simulink model "FM_V6_Zikun"  (R2022b)
settings: Solver=VariableStepAuto  StartTime=0.0  StopTime=1240
values from neighbouring files (symbols this model uses):
  A_fc = 550    [CNV.m]
  A_st = 1.1*A_fc*1E-4*n_cell*0.0012    (= 0.047553)    [CNV.m]
  A_T_rm = 0.005    [CNV.m]
  b11 = 0.005139    [CNV.m]
  b12 = 0.00326    [CNV.m]
  b2 = 350    [CNV.m]
  c1 = 10    [CNV.m]
  c3 = 2    [CNV.m]
  cc = 30    [CNV.m]
  Cd_rm = 0.0124    [CNV.m]
  Cp_air = 1005    [CNV.m]
  Cp_cl = 4180    [CNV.m]
  Cp_st = Cp_Al*1.5    (= 1350)    [CNV.m]
  F = 96485    [CNV.m]
  gamma = 1.4    [CNV.m]
  H_conv_st = 3    [CNV.m]
  i_max = 2.2    [CNV.m]
  k_ca_out = 0.2177*10^(-5)    (= 2.177e-06)    [CNV.m]
  K_sm_out = 0.3629*10^-5    (= 3.629e-06)    [CNV.m]
  kd_cp = 0.01    [CNV.m]
  kd_rm = 0    [CNV.m]
  ki_cp = 0.1    [CNV.m]
  ki_fan = -1E-5    (= -1e-05)    [CNV.m]
  ki_rm = -5E-8    (= -5e-08)    [CNV.m]
  kp_cp = 7.5    [CNV.m]
  kp_fan = -0.5    [CNV.m]
  kp_rm = -8E-7    (= -8e-07)    [CNV.m]
  M_a = 29*10^-3    (= 0.029)    [CNV.m]
  M_H2 = 2*10^-3    (= 0.002)    [CNV.m]
  m_H2_initial = P_atm*V_an/(R_H2*T_atm)    (= 0.00044494386048)    [CNV.m]
  m_H2O_initial = 0.005    [CNV.m]
  M_m_dry = 1.1    [CNV.m]
  M_N2 = 28*10^-3    (= 0.028)    [CNV.m]
  m_N2_initial = P_atm*(1-y_O2)*V_ca/(R_N2*T_atm)    (= 0.00586138039643)    [CNV.m]
  M_O2 = 32*10^-3    (= 0.032)    [CNV.m]
  m_O2_initial = P_atm*y_O2*V_ca/(R_O2*T_atm)    (= 0.00177998712422)    [CNV.m]
  m_st = n_cell*A_fc*t_m*rho_m_dry+(V_ca+V_an)*rho_Al*2.5    (= 87.4506875)    [CNV.m]
  M_v = 18*10^-3    (= 0.018)    [CNV.m]
  n_cell = 655    [CNV.m]
  P_a = P_atm*(1-L*h/T_atm)^(g*M_a/(R*L))    [CNV.m]
  P_atm = 101.25*10^3    (= 101250)    [CNV.m]
  P_ca_ref = 2.5*P_a    [CNV.m]
  phi_a = 0.1    [CNV.m]
  phi_des = 1    [CNV.m]
  R = 8.315    [CNV.m]
  R_a = 286.9    [CNV.m]
  R_H2 = 4124.3    [CNV.m]
  R_N2 = 296.8    [CNV.m]
  R_O2 = 259.8    [CNV.m]
  R_v = 461.5    [CNV.m]
  rho_a = P_a/(R_a*T_a)    [CNV.m]
  rho_H2 = 0.0899    [CNV.m]
  rho_m_dry = 0.002    [CNV.m]
  rho_N2 = 1.165    [CNV.m]
  T_a = T_atm-h*L    [CNV.m]
  T_atm = 298.15    [CNV.m]
  T_cl = 353.15    [CNV.m]
  t_m = 0.01    [CNV.m]
  T_rm = 303.15    [CNV.m]
  T_st_ref = 353.15    [CNV.m]
  V_an = n_cell*A_fc*10^(-4)*0.0005*0.3    (= 0.00540375)    [CNV.m]
  V_ca = n_cell*A_fc*10^(-4)*0.0006*0.3    (= 0.0064845)    [CNV.m]
  V_rm = 0.005    [CNV.m]
  V_sm = 0.02    [CNV.m]
  y_O2_ca_in = 0.21    [CNV.m]
libraries: fl_lib x64, nesl_utility x40, ee_lib x18, fl_ps_legacy_lib x6, SimscapeFluids_lib x5, slpidlib x4, simulink x3, batteryecm_lib x1, autolibshared x1
(part 3 of 6)

== system FM_V6_Zikun/Subsystem/Air Cooler ==
  W_sm_out : Inport
  P_sm : Inport  Port=2
  Constant : Constant  Value=P_a
  Constant1 : Constant  Value=T_a
  Constant2 : Constant  Value=phi_a
  Constant3 : Constant  Value=T_cl
  MATLAB Function : MATLAB Function  TreatAsAtomicUnit=on
  W_cl : Outport
  phi_cl : Outport  Port=2
  psat_Tcl : Outport  Port=3
  P_cl : Outport  Port=4
  T_cl : Outport  Port=5
  wires:
  P_sm/1 -> P_cl/1, MATLAB Function/1(P_cl)
  MATLAB Function/1(phi_cl) -> phi_cl/1
  MATLAB Function/2(T_cl) -> T_cl/1
  W_sm_out/1 -> W_cl/1
  MATLAB Function/3(psat_Tcl) -> psat_Tcl/1
  Constant/1 -> MATLAB Function/2(P_a)
  Constant1/1 -> MATLAB Function/3(T_a)
  Constant2/1 -> MATLAB Function/4(phi_a)
  Constant3/1 -> MATLAB Function/5("T_cl ")

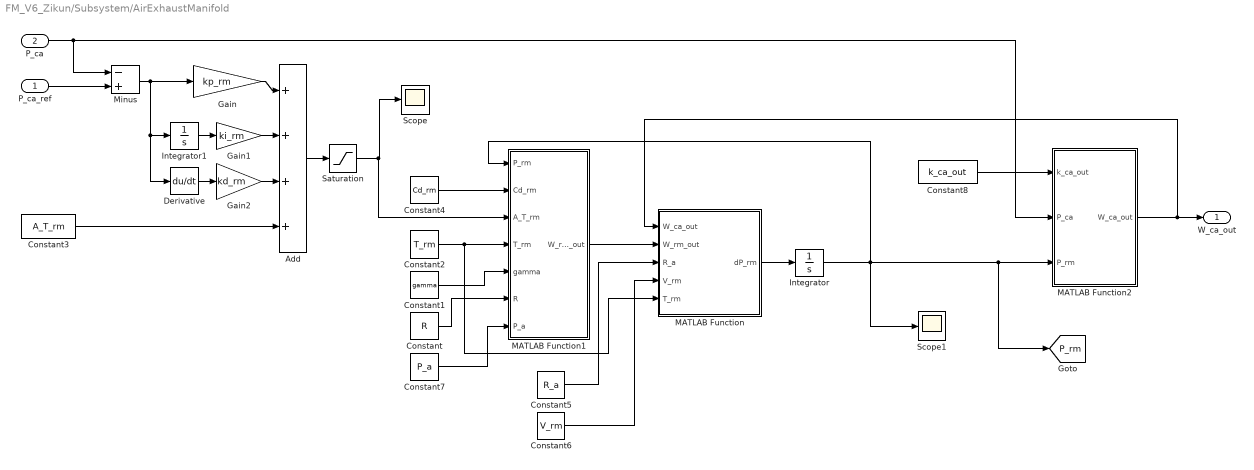
== system FM_V6_Zikun/Subsystem/AirExhaustManifold ==
  P_ca_ref : Inport
  P_ca : Inport  Port=2
  Add : Sum  Inputs=++++
  Constant : Constant  Value=R
  Constant1 : Constant  Value=gamma
  Constant2 : Constant  Value=T_rm
  Constant3 : Constant  Value=A_T_rm
  Constant4 : Constant  Value=Cd_rm
  Constant5 : Constant  Value=R_a
  Constant6 : Constant  Value=V_rm
  Constant7 : Constant  Value=P_a
  Constant8 : Constant  Value=k_ca_out
  Derivative : Derivative
  Gain : Gain  Gain=kp_rm
  Gain1 : Gain  Gain=ki_rm
  Gain2 : Gain  Gain=kd_rm
  Integrator : Integrator  InitialCondition=P_atm
  Integrator1 : Integrator
  MATLAB Function : MATLAB Function  TreatAsAtomicUnit=on
  MATLAB Function1 : MATLAB Function  TreatAsAtomicUnit=on
  MATLAB Function2 : MATLAB Function  TreatAsAtomicUnit=on
  Minus : Sum  Inputs=-+
  Saturation : Saturate  UpperLimit=0.04  LowerLimit=0
  Scope : Scope
  Scope1 : Scope
  W_ca_out : Outport
  tag scope: P_rm=global
  wires:
  MATLAB Function1/1(W_rm_out) -> MATLAB Function/2(W_rm_out)
  MATLAB Function/1(dP_rm) -> Integrator/1
  Integrator/1 -> Scope1/1, [P_rm], MATLAB Function2/3(P_rm), MATLAB Function1/1(P_rm)
  Constant/1 -> MATLAB Function1/6(R)
  Constant1/1 -> MATLAB Function1/5(gamma)
  Constant2/1 -> MATLAB Function/5(T_rm), MATLAB Function1/4(T_rm)
  Constant4/1 -> MATLAB Function1/2(Cd_rm)
  Constant5/1 -> MATLAB Function/3(R_a)
  Constant6/1 -> MATLAB Function/4(V_rm)
  Constant7/1 -> MATLAB Function1/7(P_a)
  MATLAB Function2/1(W_ca_out) -> MATLAB Function/1(W_ca_out), W_ca_out/1
  P_ca/1 -> Minus/1, MATLAB Function2/2(P_ca)
  Constant8/1 -> MATLAB Function2/1(k_ca_out)
  P_ca_ref/1 -> Minus/2
  Minus/1 -> Derivative/1, Integrator1/1, Gain/1
  Integrator1/1 -> Gain1/1
  Gain/1 -> Add/1
  Gain1/1 -> Add/2
  Constant3/1 -> Add/4
  Derivative/1 -> Gain2/1
  Gain2/1 -> Add/3
  Add/1 -> Saturation/1
  Saturation/1 -> MATLAB Function1/3(A_T_rm), Scope/1

== system FM_V6_Zikun/Subsystem/Blower ==
  P_an_in : Inport
  lambda_H2 : Inport  Port=2
  ny_blower : Inport  Port=3
  W_H2_tank : Inport  Port=4
  P_an : Inport  Port=5
  H2_ratio : Inport  Port=6
  Constant : Constant  Value=rho_H2
  Constant1 : Constant  Value=rho_N2
  MATLAB Function : MATLAB Function  TreatAsAtomicUnit=on
  W_an_in : Outport
  W_an_out : Outport  Port=2
  P_blower : Outport  Port=3
  wires:
  lambda_H2/1 -> MATLAB Function/4(lambda_H2)
  H2_ratio/1 -> MATLAB Function/6(H2_ratio)
  ny_blower/1 -> MATLAB Function/5(ny_blower)
  W_H2_tank/1 -> MATLAB Function/3(W_H2_tank)
  Constant/1 -> MATLAB Function/2(rho_N2)
  Constant1/1 -> MATLAB Function/1(rho_H2)
  MATLAB Function/1(W_an_in) -> W_an_in/1
  MATLAB Function/2(W_an_out) -> W_an_out/1
  MATLAB Function/3(P_blower) -> P_blower/1
  P_an/1 -> MATLAB Function/8(P_an)
  P_an_in/1 -> MATLAB Function/7(P_an_in)

== system FM_V6_Zikun/Subsystem/Compressor ==
  I_st : Inport
  P_ca : Inport  Port=2
  P_sm : Inport  Port=3
  Abs : Abs  ZeroCross=off  SaturateOnIntegerOverflow=off
  Add : Sum  Inputs=+-
  Constant2 : Constant
  Constant6 : Constant  Value=T_a
  Constant7 : Constant  Value=P_a
  Display : Display
  Divide : Product  Inputs=*/
  Divide1 : Product  Inputs=**
  Power calc 2 : Subsystem
      settings: PortSchema="{\"entries\":[{\"content\":{\"sides\":[{\"content\":{\"connectorIds\":[\"In1\",\"In2\",\"In3\"]},\"type\":\"ConnectorPlacement.EquallySpacedRectSide\",\"uuid\":\"8b079436-ea2a-4c47-8bc6-4d08a6a8278c\"},{\"content\":{\"connectorIds\":[\"In4\",\"Out1\"],\"side\":\"RIGHT\"},\"type\":\"ConnectorPlacement.EquallySpacedRectSide\",\"uuid\":\"2ad3baf7-33f6-4d58-a512-a1947502cd3d\"},{\"content\":{\"connectorIds\":[],\"side\":\"TOP\"},\"type\":\"ConnectorPlacement.EquallySpacedRectSide\",\"uuid\":\"d6297fa1-7292-4bed-8060-dba2913c02c2\"}]},\"type\":\"ConnectorPlacement.EquallySpacedConnector\",\"uuid\":\"103abd89-9500-4b01-83b0-a840418a3fc8\"}],\"packageUris\":[\"http://schema.mathworks.com/mf0/Connector/R2020b\"],\"version\":\"1.0\"}"
  Saturation : Saturate  UpperLimit=0.2  LowerLimit=4e-3  ZeroCross=off
  Scope : Scope
  Scope1 : Scope
  Subsystem : Subsystem
  Temperature of the air leaving the compressor (2.8) : Subsystem
  maximum efficiency of compressor : Constant  Value=0.9
  "rate of specific heats of air " : Constant  Value=gamma
  W_cp : Outport
  T_cp_out : Outport  Port=2
  Power_cp_them : Outport  Port=3
  Power_cp_tot : Outport  Port=4
  wires:
  "rate of specific heats of air "/1 -> Power calc 2/3(gamma), Temperature of the air leaving the compressor (2.8)/5(gamma)
  Constant6/1 -> Temperature of the air leaving the compressor (2.8)/1(T_atm)
  maximum efficiency of compressor/1 -> Add/2, Divide/2, Temperature of the air leaving the compressor (2.8)/2(eta_cp)
  Temperature of the air leaving the compressor (2.8)/1(T_cp_out) -> T_cp_out/1
  Constant7/1 -> Power calc 2/2(P_cp_in), Temperature of the air leaving the compressor (2.8)/4(P_atm)
  I_st/1 -> Subsystem/2(I_st)
  Power calc 2/1(Power_cp) -> Divide/1
  Divide/1 -> Abs/1
  Constant2/1 -> Add/1
  Add/1 -> Divide1/2
  Divide1/1 -> Power_cp_them/1
  Abs/1 -> Divide1/1, Display/1, Power_cp_tot/1
  [W_O2_ca_in] -> Subsystem/1(W_O2_ca_in)
  P_ca/1 -> Subsystem/3(P_ca)
  P_sm/1 -> Power calc 2/1(P_cp_out), Temperature of the air leaving the compressor (2.8)/3(P_sm)
  Subsystem/1(W_cp) -> Saturation/1
  Saturation/1 -> Scope/1, W_cp/1, Scope1/1, Power calc 2/4(W_cp_in)

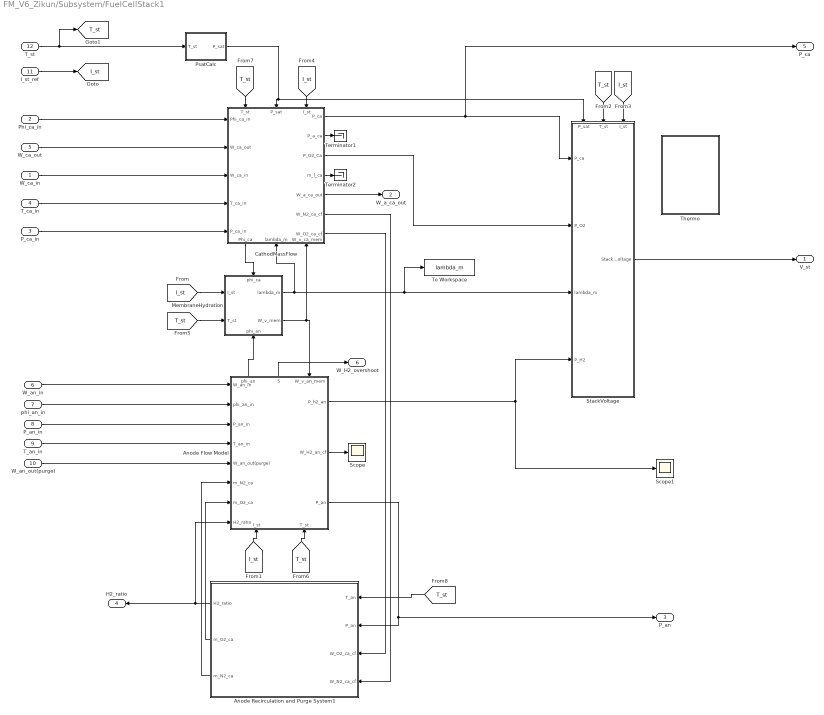
== system FM_V6_Zikun/Subsystem/FuelCellStack1 ==
  W_ca_in : Inport
  Phi_ca_in : Inport  Port=2
  P_ca_in : Inport  Port=3
  T_ca_in : Inport  Port=4
  W_ca_out : Inport  Port=5
  W_an_in : Inport  Port=6
  phi_an_in : Inport  Port=7
  P_an_in : Inport  Port=8
  T_an_in : Inport  Port=9
  W_an_out(purge) : Inport  Port=10
  I_st_ref : Inport  Port=11
  T_st : Inport  Port=12
  Anode Flow Model : Subsystem
      settings: PortSchema="{\"entries\":[{\"content\":{\"sides\":[{\"content\":{\"connectorIds\":[\"In1\",\"In2\",\"In3\",\"In4\",\"In5\",\"In6\",\"In7\",\"In8\"]},\"type\":\"ConnectorPlacement.EquallySpacedRectSide\",\"uuid\":\"477fe13c-ae2c-434a-aa62-6a7137066034\"},{\"content\":{\"connectorIds\":[\"Out1\",\"Out2\",\"Out3\"],\"side\":\"RIGHT\"},\"type\":\"ConnectorPlacement.EquallySpacedRectSide\",\"uuid\":\"66550877-05b9-4d53-a95b-0d13dddd1ae9\"},{\"content\":{\"connectorIds\":[\"Out4\",\"Out5\",\"In9\"],\"side\":\"TOP\"},\"type\":\"ConnectorPlacement.EquallySpacedRectSide\",\"uuid\":\"dee2e959-3be9-4270-9608-f17df99829af\"},{\"content\":{\"connectorIds\":[\"In10\",\"In11\"],\"side\":\"BOTTOM\"},\"type\":\"ConnectorPlacement.EquallySpacedRectSide\",\"uuid\":\"e68932cb-a3ca-49aa-99ac-394e109cb21d\"}]},\"type\":\"ConnectorPlacement.EquallySpacedConnector\",\"uuid\":\"e53fddc6-f473-4a61-b934-687e83f91b65\"}],\"packageUris\":[\"http://schema.mathworks.com/mf0/Connector/R2020b\"],\"version\":\"1.0\"}"
  Anode Recirculation and Purge System1 : Subsystem
      settings: PortSchema="{\"entries\":[{\"content\":{\"sides\":[{\"content\":{\"connectorIds\":[\"Out1\",\"Out2\",\"Out3\"]},\"type\":\"ConnectorPlacement.EquallySpacedRectSide\",\"uuid\":\"a717ff69-9a06-432a-8ec9-0b41de582fa8\"},{\"content\":{\"connectorIds\":[\"In1\",\"In2\",\"In3\",\"In4\"],\"side\":\"RIGHT\"},\"type\":\"ConnectorPlacement.EquallySpacedRectSide\",\"uuid\":\"e2c7096e-75de-462f-89fb-70e142ee793c\"},{\"content\":{\"connectorIds\":[],\"side\":\"TOP\"},\"type\":\"ConnectorPlacement.EquallySpacedRectSide\",\"uuid\":\"2426b314-6327-4045-9254-2b33a242dd4e\"},{\"content\":{\"connectorIds\":[],\"side\":\"BOTTOM\"},\"type\":\"ConnectorPlacement.EquallySpacedRectSide\",\"uuid\":\"28581630-fccf-4c59-a85b-fca9f25db1df\"}]},\"type\":\"ConnectorPlacement.EquallySpacedConnector\",\"uuid\":\"c799c0e9-037d-437b-b392-b2fa1dfcad00\"}],\"packageUris\":[\"http://schema.mathworks.com/mf0/Connector/R2020b\"],\"version\":\"1.0\"}"
  CathodMassFlow : Subsystem
      settings: PortSchema="{\"entries\":[{\"content\":{\"sides\":[{\"content\":{\"connectorIds\":[\"In1\",\"In2\",\"In3\",\"In4\",\"In5\"]},\"type\":\"ConnectorPlacement.EquallySpacedRectSide\",\"uuid\":\"a5816526-b2df-4ff7-b309-d39278f05798\"},{\"content\":{\"connectorIds\":[\"Out1\",\"Out2\",\"Out3\",\"Out4\",\"Out5\",\"Out6\",\"Out7\"],\"side\":\"RIGHT\"},\"type\":\"ConnectorPlacement.EquallySpacedRectSide\",\"uuid\":\"a3a8a0b8-4f26-4d97-8833-d547d26a82ce\"},{\"content\":{\"connectorIds\":[\"In6\",\"In7\",\"In8\"],\"side\":\"TOP\"},\"type\":\"ConnectorPlacement.EquallySpacedRectSide\",\"uuid\":\"a0145b7a-873e-4436-80c5-f848de3e3117\"},{\"content\":{\"connectorIds\":[\"Out8\",\"In9\",\"In10\"],\"side\":\"BOTTOM\"},\"type\":\"ConnectorPlacement.EquallySpacedRectSide\",\"uuid\":\"3c36750c-8b40-4a1a-a95d-a988a8ace63a\"}]},\"type\":\"ConnectorPlacement.EquallySpacedConnector\",\"uuid\":\"934b3933-c5aa-40b8-8fa9-71f43b151d81\"}],\"packageUris\":[\"http://schema.mathworks.com/mf0/Connector/R2020b\"],\"version\":\"1.0\"}"
  MembraneHydration : Subsystem
      settings: PortSchema="{\"entries\":[{\"content\":{\"sides\":[{\"content\":{\"connectorIds\":[\"In1\",\"In2\"]},\"type\":\"ConnectorPlacement.EquallySpacedRectSide\",\"uuid\":\"3fc204c3-9c69-492e-9375-472aea363e1b\"},{\"content\":{\"connectorIds\":[\"Out1\",\"Out2\"],\"side\":\"RIGHT\"},\"type\":\"ConnectorPlacement.EquallySpacedRectSide\",\"uuid\":\"92fcb20f-c63d-4632-a8b2-72361d3984f2\"},{\"content\":{\"connectorIds\":[\"In3\"],\"side\":\"TOP\"},\"type\":\"ConnectorPlacement.EquallySpacedRectSide\",\"uuid\":\"2bf67bc3-afc1-4ec2-8a6f-f1995431a2a1\"},{\"content\":{\"connectorIds\":[\"In4\"],\"side\":\"BOTTOM\"},\"type\":\"ConnectorPlacement.EquallySpacedRectSide\",\"uuid\":\"b4bf2ddb-e361-4582-99a1-8ca6e4cff378\"}]},\"type\":\"ConnectorPlacement.EquallySpacedConnector\",\"uuid\":\"9ca90662-d7f0-47d0-8eb8-23aab38cb896\"}],\"packageUris\":[\"http://schema.mathworks.com/mf0/Connector/R2020b\"],\"version\":\"1.0\"}"
  PsatCalc : MATLAB Function  TreatAsAtomicUnit=on
  Scope : Scope
  Scope1 : Scope
  StackVoltage : Subsystem
      settings: PortSchema="{\"entries\":[{\"content\":{\"sides\":[{\"content\":{\"connectorIds\":[\"In1\",\"In2\",\"In3\",\"In4\"]},\"type\":\"ConnectorPlacement.EquallySpacedRectSide\",\"uuid\":\"31c21434-8ccd-4c9e-84e7-d59d7b2b32c9\"},{\"content\":{\"connectorIds\":[\"Out1\"],\"side\":\"RIGHT\"},\"type\":\"ConnectorPlacement.EquallySpacedRectSide\",\"uuid\":\"a03264e4-aeb3-4f9b-a3b2-cfddd05e7880\"},{\"content\":{\"connectorIds\":[\"In5\",\"In6\",\"In7\"],\"side\":\"TOP\"},\"type\":\"ConnectorPlacement.EquallySpacedRectSide\",\"uuid\":\"8542eea2-4f96-46a3-8a8b-d86d68868d64\"}]},\"type\":\"ConnectorPlacement.EquallySpacedConnector\",\"uuid\":\"2ea05213-dddc-4bd5-a30f-0985ad8bd6f4\"}],\"packageUris\":[\"http://schema.mathworks.com/mf0/Connector/R2020b\"],\"version\":\"1.0\"}"
  Terminator1 : Terminator
  Terminator2 : Terminator
  Thermo : Subsystem
  To Workspace : ToWorkspace  VariableName=lambda_m  SaveFormat=Timeseries  SampleTime=-1
  V_st : Outport
  W_a_ca_out : Outport  Port=2
  P_an : Outport  Port=3
  H2_ratio : Outport  Port=4
  P_ca : Outport  Port=5
  W_H2_overshoot : Outport  Port=6
  tag scope: I_st=global, T_st=global
  wires:
  CathodMassFlow/1(P_ca) -> P_ca/1, StackVoltage/1(P_ca)
  CathodMassFlow/3(P_O2_Ca) -> StackVoltage/2(P_O2)
  CathodMassFlow/8(Phi_ca) -> MembraneHydration/3(phi_ca)
  Anode Flow Model/4(phi_an) -> MembraneHydration/4(phi_an)
  MembraneHydration/2(W_v_mem) -> CathodMassFlow/10(W_v_ca_mem), Anode Flow Model/9(W_v_an_mem)
  MembraneHydration/1(lambda_m) -> CathodMassFlow/9(lambda_m), To Workspace/1, StackVoltage/3(lambda_m)
  Anode Flow Model/1(P_h2_an) -> StackVoltage/4(P_H2), Scope1/1
  CathodMassFlow/5(W_a_ca_out) -> W_a_ca_out/1
  W_ca_in/1 -> CathodMassFlow/3(W_ca_in)
  W_ca_out/1 -> CathodMassFlow/2(W_ca_out)
  Phi_ca_in/1 -> CathodMassFlow/1(Phi_ca_in)
  W_an_in/1 -> Anode Flow Model/1(W_an_in)
  phi_an_in/1 -> Anode Flow Model/2(phi_an_in)
  P_an_in/1 -> Anode Flow Model/3(P_an_in)
  T_an_in/1 -> Anode Flow Model/4(T_an_in)
  CathodMassFlow/2(P_a_ca) -> Terminator1/1
  CathodMassFlow/4(m_l_ca) -> Terminator2/1
  T_ca_in/1 -> CathodMassFlow/4(T_ca_in)
  P_ca_in/1 -> CathodMassFlow/5(P_ca_in)
  T_st/1 -> [T_st], PsatCalc/1(T_st)
  I_st_ref/1 -> [I_st]
  [I_st] -> MembraneHydration/1(I_st)
  [I_st] -> Anode Flow Model/10(I_st)
  [I_st] -> StackVoltage/7(I_st)
  [I_st] -> CathodMassFlow/8(I_st)
  [T_st] -> CathodMassFlow/6(T_st)
  [T_st] -> StackVoltage/6(T_st)
  [T_st] -> Anode Flow Model/11(T_st)
  [T_st] -> MembraneHydration/2(T_st)
  CathodMassFlow/6(W_N2_ca_cf) -> Anode Recirculation and Purge System1/4(W_N2_ca_cf)
  CathodMassFlow/7(W_O2_ca_cf) -> Anode Recirculation and Purge System1/3(W_O2_ca_cf)
  W_an_out(purge)/1 -> Anode Flow Model/5(W_an_out(purge))
  Anode Recirculation and Purge System1/1(H2_ratio) -> Anode Flow Model/8(H2_ratio), H2_ratio/1
  Anode Recirculation and Purge System1/3(m_N2_ca) -> Anode Flow Model/6(m_N2_ca)
  Anode Recirculation and Purge System1/2(m_O2_ca) -> Anode Flow Model/7(m_O2_ca)
  Anode Flow Model/2(W_H2_an_cf) -> Scope/1
  [T_st] -> Anode Recirculation and Purge System1/1(T_an)
  PsatCalc/1(P_sat) -> CathodMassFlow/7(P_sat), StackVoltage/5(P_sat)
  StackVoltage/1(StackVoltage) -> V_st/1
  Anode Flow Model/5(W_H2_overshoot) -> W_H2_overshoot/1
  Anode Flow Model/3(P_an) -> P_an/1, Anode Recirculation and Purge System1/2(P_an)

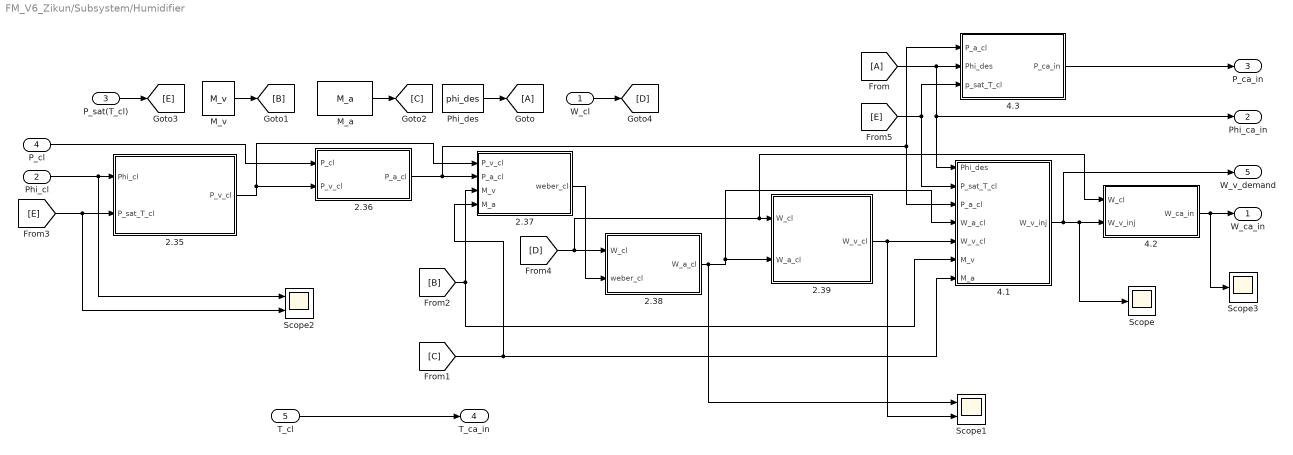
== system FM_V6_Zikun/Subsystem/Humidifier ==
  W_cl : Inport
  Phi_cl : Inport  Port=2
  P_sat(T_cl) : Inport  Port=3
  P_cl : Inport  Port=4
  T_cl : Inport  Port=5
  2.35 : MATLAB Function  TreatAsAtomicUnit=on
  2.36 : MATLAB Function  TreatAsAtomicUnit=on
  2.37 : MATLAB Function  TreatAsAtomicUnit=on
  2.38 : MATLAB Function  TreatAsAtomicUnit=on
  2.39 : MATLAB Function  TreatAsAtomicUnit=on
  4.1 : MATLAB Function  TreatAsAtomicUnit=on
  4.2 : MATLAB Function  TreatAsAtomicUnit=on
  4.3 : MATLAB Function  TreatAsAtomicUnit=on
  From : From
  Goto : Goto
  M_a : Constant  Value=M_a
  M_v : Constant  Value=M_v
  Phi_des : Constant  Value=phi_des
  Scope : Scope
  Scope1 : Scope  NumInputPorts=2
  Scope2 : Scope  NumInputPorts=2
  Scope3 : Scope
  W_ca_in : Outport
  Phi_ca_in : Outport  Port=2
  P_ca_in : Outport  Port=3
  T_ca_in : Outport  Port=4
  W_v_demand : Outport  Port=5
  wires:
  4.3/1(P_ca_in) -> P_ca_in/1
  4.1/1(W_v_inj) -> Scope/1, 4.2/2(W_v_inj), W_v_demand/1
  2.36/1(P_a_cl) -> 4.1/3(P_a_cl), 4.3/1(P_a_cl), 2.37/2(P_a_cl)
  2.39/1(W_v_cl) -> Scope1/2, 4.1/5(W_v_cl)
  2.38/1(W_a_cl) -> Scope1/1, 2.39/2(W_a_cl), 4.1/4(W_a_cl)
  2.35/1(P_v_cl) -> 2.37/1(P_v_cl), 2.36/2(P_v_cl)
  Phi_cl/1 -> Scope2/1, 2.35/1(Phi_cl)
  P_cl/1 -> 2.36/1(P_cl)
  Phi_des/1 -> Goto/1
  M_v/1 -> [B]
  M_a/1 -> [C]
  2.37/1(weber_cl) -> 2.38/2(weber_cl)
  P_sat(T_cl)/1 -> [E]
  [E] -> Scope2/2, 2.35/2(P_sat_T_cl)
  W_cl/1 -> [D]
  From/1 -> Phi_ca_in/1, 4.1/1(Phi_des), 4.3/2(Phi_des)
  [B] -> 4.1/6(M_v), 2.37/3(M_v)
  [C] -> 4.1/7(M_a), 2.37/4(M_a)
  [D] -> 4.2/1(W_cl), 2.39/1(W_cl), 2.38/1(W_cl)
  [E] -> 4.3/3(p_sat_T_cl), 4.1/2(P_sat_T_cl)
  T_cl/1 -> T_ca_in/1
  4.2/1(W_ca_in) -> Scope3/1, W_ca_in/1

== system FM_V6_Zikun/Subsystem/Hydrogen Tank // Hydrogen Valve // Regulator1 ==
  Tank Volume : Inport
  Initial Tank Pressure : Inport  Port=2
  Tank Temperature : Inport  Port=3
  Regulator Anode Pressure : Inport  Port=4
  P_an : Inport  Port=5
  Constant : Constant  Value=R_H2
  Gain : Gain  Gain=1/M_N2
  Integrator : Integrator
  MATLAB Function1 : MATLAB Function  TreatAsAtomicUnit=on
  PID Controller : slpidlib/PID Controller  Controller=PI  Form=Parallel  TimeDomain=Continuous-time  UseExternalTs=off  SampleTime=-1  IntegratorMethod=Forward Euler  FilterMethod=Forward Euler  ControllerParametersSource=internal  P=6e-7  I=0  UseKiTs=off  D=0  N=100  UseFilter=on  TunerSelectOption=Transfer Function Based (PID Tuner App)  InitialConditionSource=internal  InitialConditionForIntegrator=0  InitialConditionForFilter=0  DifferentiatorICPrevScaledInput=0  ExternalReset=none  TrackingMode=off  Kt=1  LimitOutput=on  SatLimitsSource=internal  UpperSaturationLimit=0.005  LowerSaturationLimit=-0.04  LinearizeAsGain=on  AntiWindupMode=none  Kb=1  LimitIntegrator=off  UpperIntegratorSaturationLimit=inf  LowerIntegratorSaturationLimit=-inf  POutMin=[]  POutMax=[]  IOutMin=[]  IOutMax=[]  DOutMin=[]  DOutMax=[]  NOutMin=[]  NOutMax=[]  SumOutMin=[]  SumOutMax=[]  SaturationOutMin=[]  SaturationOutMax=[]  PParamMin=[]  PParamMax=[]  IParamMin=[]  IParamMax=[]  DParamMin=[]  DParamMax=[]  NParamMin=[]  NParamMax=[]  KbParamMin=[]  KbParamMax=[]  KtParamMin=[]  KtParamMax=[]  KbOutMin=[]  KbOutMax=[]  KtOutMin=[]  KtOutMax=[]  IntegratorOutMin=[]  IntegratorOutMax=[]  FilterOutMin=[]  FilterOutMax=[]  SumI1OutMin=[]  SumI1OutMax=[]  SumI2OutMin=[]  SumI2OutMax=[]  SumI3OutMin=[]  SumI3OutMax=[]  SumI4OutMin=[]  SumI4OutMax=[]  SumDOutMin=[]  SumDOutMax=[]  DifferentiatorOutMin=[]  DifferentiatorOutMax=[]  FilterDiffOutCoefMin=[]  FilterDiffOutCoefMax=[]  ReciprocalOutMin=[]  ReciprocalOutMax=[]  SumDenOutMin=[]  SumDenOutMax=[]  SumNumOutMin=[]  SumNumOutMax=[]  DivideOutMin=[]  DivideOutMax=[]  UdiffTsProdOutMin=[]  UdiffTsProdOutMax=[]  NTsProdOutMin=[]  NTsProdOutMax=[]  UintegralTsProdOutMin=[]  UintegralTsProdOutMax=[]  UngainTsProdOutMin=[]  UngainTsProdOutMax=[]  ClampingZeroOutDataTypeStr=Inherit: Inherit via back propagation  ClampingZeroOutMin=[]  ClampingZeroOutMax=[]  FilterDenConstantOutDataTypeStr=Inherit: Inherit via back propagation  FilterDenConstantOutMin=[]  FilterDenConstantOutMax=[]  PCopyOutDataTypeStr=Inherit: Inherit via back propagation  PCopyOutMin=[]  PCopyOutMax=[]  NCopyOutDataTypeStr=Inherit: Inherit via back propagation  NCopyOutMin=[]  NCopyOutMax=[]  IntegratorContinuousStateAttributes=''  IntegratorStateMustResolveToSignalObject=off  IntegratorRTWStateStorageClass=Auto  FilterContinuousStateAttributes=''  FilterStateMustResolveToSignalObject=off  FilterRTWStateStorageClass=Auto  ParallelPVariant=InternalParameters  IdealPVariant=Disabled  IVariant=InternalParameters  DVariant=Disabled  IntegratorVariant=Continuous  SatVariant=Enabled  AWVariant=Passthrough  PCopyVariant=Disabled  TRVariant=Disabled  FdbkBlocksVariant=Forward  IdealPFdbkVariant=Disabled  SatFdbkVariant=Disabled  DerivativeFilterVariant=Disabled  NVariant=Disabled  NCopyVariant=Disabled_SignalSpec  FilterICVariant=Disabled  IntegratorICVariant=InternalICs  ExternalResetVariant=Disabled  TRSumVariant=Passthrough  SumFdbkVariant=Disabled  SumVariant=Sum_PI  TsampFilterVariant=InternalTs  TsampNgainVariant=Passthrough  TsampIntegralVariant=Passthrough  ExternalSaturationOutDataTypeStr=Inherit: Same as second input
  Scope : Scope
  Subtract : Sum  Inputs=+-
  P_tank : Outport
  W_H2_tank : Outport  Port=2
  wires:
  P_an/1 -> Subtract/2
  Regulator Anode Pressure/1 -> Subtract/1
  Integrator/1 -> Gain/1
  Gain/1 -> MATLAB Function1/5(n_consumed)
  Tank Volume/1 -> MATLAB Function1/2(V_tank)
  Tank Temperature/1 -> MATLAB Function1/3(T_tank)
  Initial Tank Pressure/1 -> MATLAB Function1/4(P_tank_nom)
  Constant/1 -> MATLAB Function1/1(R_H2)
  MATLAB Function1/1(P_tank) -> P_tank/1
  Subtract/1 -> PID Controller/1
  PID Controller/1 -> Scope/1, Integrator/1, W_H2_tank/1

== system FM_V6_Zikun/Subsystem/Subsystem ==
  W_H2_Tank : Inport
  P_an : Inport  Port=2
  Add : Sum  Inputs=+-
  Add1 : Sum  Inputs=+-
  Constant : Constant  Value=R_H2
  Constant1 : Constant  Value=T_a
  Constant2 : Constant  Value=1*10^-3
  Gain : Gain  Gain=1e-8
  Integrator : Integrator  InitialCondition=1e-4
  MATLAB Function : MATLAB Function  TreatAsAtomicUnit=on
  Scope : Scope
  Scope1 : Scope
  W_H2_manifold : Outport
  wires:
  Constant/1 -> MATLAB Function/2(R_H2)
  Constant1/1 -> MATLAB Function/3(T_rm)
  Constant2/1 -> MATLAB Function/4(V_H2_manifold)
  MATLAB Function/1(P_H2_manifold) -> Add/1
  P_an/1 -> Add/2
  Add/1 -> Gain/1
  Gain/1 -> Add1/2, Scope/1, W_H2_manifold/1
  Integrator/1 -> MATLAB Function/1(m_H2), Scope1/1
  W_H2_Tank/1 -> Add1/1
  Add1/1 -> Integrator/1

== system FM_V6_Zikun/Subsystem/Subsystem2 ==
  I_st : Inport
  P_st : Inport  Port=2
  Subsystem : Subsystem
  ThermoCalc : Subsystem
  T_st : Outport
  P_tot : Outport  Port=2
  P_fan_loss : Outport  Port=3
  P_pump_loss : Outport  Port=4
  wires:
  ThermoCalc/1(T_st) -> Subsystem/1(T_cl_in), T_st/1
  P_st/1 -> ThermoCalc/2(P_st)
  I_st/1 -> Subsystem/2(I_st), ThermoCalc/1(I_st)
  Subsystem/3(P_cl) -> ThermoCalc/3(P_cl)
  Subsystem/1(P_pump_loss) -> P_pump_loss/1
  Subsystem/2(P_fan_loss) -> P_fan_loss/1
  ThermoCalc/2(P_tot_st) -> P_tot/1

== system FM_V6_Zikun/Subsystem/Supply Manifold ==
  W_cp : Inport
  T_cp_out : Inport  Port=2
  P_ca : Inport  Port=3
  Manifold Filling : Subsystem
      settings: PortSchema="{\"entries\":[{\"content\":{\"sides\":[{\"content\":{\"connectorIds\":[\"In1\",\"In2\"]},\"type\":\"ConnectorPlacement.EquallySpacedRectSide\",\"uuid\":\"5b708061-f651-4e95-ab82-a4e5a10c41aa\"},{\"content\":{\"connectorIds\":[],\"side\":\"RIGHT\"},\"type\":\"ConnectorPlacement.EquallySpacedRectSide\",\"uuid\":\"45f2c177-5321-40a9-9b70-6a6ced21c730\"},{\"content\":{\"connectorIds\":[],\"side\":\"TOP\"},\"type\":\"ConnectorPlacement.EquallySpacedRectSide\",\"uuid\":\"ee9f469e-0be0-432d-ad01-7aba5a85248f\"},{\"content\":{\"connectorIds\":[\"Out1\",\"Out2\",\"In3\"],\"side\":\"BOTTOM\"},\"type\":\"ConnectorPlacement.EquallySpacedRectSide\",\"uuid\":\"36fd777e-57dd-45d2-bfa2-d5269b7bf5c5\"}]},\"type\":\"ConnectorPlacement.EquallySpacedConnector\",\"uuid\":\"e32288af-c3d9-443b-a6e9-38324f9252c2\"}],\"packageUris\":[\"http://schema.mathworks.com/mf0/Connector/R2020b\"],\"version\":\"1.0\"}"
  Nozzle : Subsystem
      settings: PortSchema="{\"entries\":[{\"content\":{\"sides\":[{\"content\":{\"connectorIds\":[\"In1\"]},\"type\":\"ConnectorPlacement.EquallySpacedRectSide\",\"uuid\":\"5777e37f-23fb-4f15-af78-9892d3d66602\"},{\"content\":{\"connectorIds\":[],\"side\":\"RIGHT\"},\"type\":\"ConnectorPlacement.EquallySpacedRectSide\",\"uuid\":\"6b20c729-b7c3-4bc6-b5e0-0939bc80540e\"},{\"content\":{\"connectorIds\":[\"In2\",\"Out1\"],\"side\":\"TOP\"},\"type\":\"ConnectorPlacement.EquallySpacedRectSide\",\"uuid\":\"7214889f-27be-4955-bc42-e5ef8cefdc7b\"}]},\"type\":\"ConnectorPlacement.EquallySpacedConnector\",\"uuid\":\"587654f3-6bd3-42f6-b028-b1e2be83784f\"}],\"packageUris\":[\"http://schema.mathworks.com/mf0/Connector/R2020b\"],\"version\":\"1.0\"}"
  W_sm_out : Outport
  P_sm : Outport  Port=2
  T_sm : Outport  Port=3
  wires:
  W_cp/1 -> Manifold Filling/1(W_cp)
  T_cp_out/1 -> Manifold Filling/2(T_cp_out)
  Manifold Filling/2(T_sm) -> T_sm/1
  P_ca/1 -> Nozzle/1(P_ca)
  Nozzle/1(W_sm_out) -> W_sm_out/1, Manifold Filling/3(W_sm_out)
  Manifold Filling/1(p_sm) -> P_sm/1, Nozzle/2(P_sm)

== system FM_V6_Zikun/Subsystem/Tank ==
  W_v_ca_out : Inport
  W_v_demand : Inport  Port=2
  Integrator : Integrator  ExternalReset=rising  InitialCondition=5
  MATLAB Function : MATLAB Function  TreatAsAtomicUnit=on
  Scope : Scope
  Sum : Sum  Inputs=-+|
  Unit Delay : UnitDelay  SampleTime=-1  HasFrameUpgradeWarning=on
  m_w_tank : Outport
  wires:
  Sum/1 -> Integrator/1
  W_v_ca_out/1 -> Sum/2
  W_v_demand/1 -> Sum/1
  MATLAB Function/1(cmd_refill) -> Integrator/2
  Integrator/1 -> Unit Delay/1, m_w_tank/1, Scope/1
  Unit Delay/1 -> MATLAB Function/1(m_w_tank)

== system FM_V6_Zikun/D/Battery/Calculations ==
  " W to kW " : Gain  Gain=1/1000
  Divide : Product  Inputs=*/
  Gain : Gain  Gain=1e-3
  I^2 : fl_ps_legacy_lib/Legacy Physical Signals/Functions/PS Product
  PS-Simulink Converter : nesl_utility/PS-Simulink Converter  PhysicalDomain=network_engine_domain  SubClassName=ps_output  LeftPortType=input  RightPortType=output  PseudoPeriodic=off  Frequencies=[]  VectorFormat=1-D array  Unit=W  AffineConversion=off
  PS-Simulink Converter4 : nesl_utility/PS-Simulink Converter  PhysicalDomain=network_engine_domain  SubClassName=ps_output  LeftPortType=input  RightPortType=output  PseudoPeriodic=off  Frequencies=[]  VectorFormat=1-D array  Unit=N*m  AffineConversion=off
  Power : fl_ps_legacy_lib/Legacy Physical Signals/Functions/PS Product
  R : fl_ps_legacy_lib/Legacy Physical Signals/Functions/PS Gain  gain=0.05
  Subtract : Sum  Inputs=+-
  W to kW : Gain  Gain=1/1000
  V : PMIOPort  Side=Left
  I : PMIOPort  Port=2  Side=Left
  eff_bat : Outport
  Power_Battery : Outport  Port=2
  tag scope: Pe_battery=global, Ploss_battery=global
  wires:
  PS-Simulink Converter/1 -> W to kW/1  "Battery power"
  W to kW/1 -> Gain/1, Subtract/1, Divide/2, [Pe_battery]  "Battery"
  PS-Simulink Converter4/1 -> " W to kW "/1
  Divide/1 -> eff_bat/1
  " W to kW "/1 -> Subtract/2, [Ploss_battery]
  Subtract/1 -> Divide/1
  Gain/1 -> Power_Battery/1
  connections:
  Power/RConn1 -- PS-Simulink Converter/LConn1
  V/RConn1 -- Power/LConn1
  Power/LConn2 -- I/RConn1 -- I^2/LConn2 -- I^2/LConn1
  I^2/RConn1 -- R/LConn1
  R/RConn1 -- PS-Simulink Converter4/LConn1

== system FM_V6_Zikun/D/Motor/Electrical Power ==
  " W to kW " : Gain  Gain=1/1000
  Current Sensor : fl_lib/Electrical/Electrical Sensors/Current Sensor
  PS Product : fl_ps_legacy_lib/Legacy Physical Signals/Functions/PS Product
  PS-Simulink Converter : nesl_utility/PS-Simulink Converter  PhysicalDomain=network_engine_domain  SubClassName=ps_output  LeftPortType=input  RightPortType=output  PseudoPeriodic=off  Frequencies=[]  VectorFormat=inherit  Unit=inherit  AffineConversion=off
  PS-Simulink Converter1 : nesl_utility/PS-Simulink Converter  PhysicalDomain=network_engine_domain  SubClassName=ps_output  LeftPortType=input  RightPortType=output  PseudoPeriodic=off  Frequencies=[]  VectorFormat=inherit  Unit=inherit  AffineConversion=off
  PS-Simulink Converter3 : nesl_utility/PS-Simulink Converter  PhysicalDomain=network_engine_domain  SubClassName=ps_output  LeftPortType=input  RightPortType=output  PseudoPeriodic=off  Frequencies=[]  VectorFormat=1-D array  Unit=W  AffineConversion=off
  Scope : Scope
  Scope1 : Scope
  Voltage Sensor : fl_lib/Electrical/Electrical Sensors/Voltage Sensor
  + : PMIOPort  Side=Left
  0v : PMIOPort  Port=2  Side=Left
  - : PMIOPort  Port=3  Side=Right
  Pe_motor : Outport
  tag scope: Pe_motor=global
  wires:
  PS-Simulink Converter3/1 -> " W to kW "/1
  " W to kW "/1 -> Pe_motor/1, [Pe_motor]
  PS-Simulink Converter1/1 -> Scope1/1
  PS-Simulink Converter/1 -> Scope/1
  connections:
  Current Sensor/RConn1 -- PS-Simulink Converter1/LConn1 -- PS Product/LConn1
  -/RConn1 -- Current Sensor/RConn2 -- Voltage Sensor/LConn1
  0v/RConn1 -- Voltage Sensor/RConn2
  Voltage Sensor/RConn1 -- PS-Simulink Converter/LConn1 -- PS Product/LConn2
  PS Product/RConn1 -- PS-Simulink Converter3/LConn1
  Current Sensor/LConn1 -- +/RConn1

== system FM_V6_Zikun/D/Motor/Mechanical Power ==
  " W to kW " : Gain  Gain=1/1000
  PS Product : fl_ps_legacy_lib/Legacy Physical Signals/Functions/PS Product
  PS-Simulink Converter3 : nesl_utility/PS-Simulink Converter  PhysicalDomain=network_engine_domain  SubClassName=ps_output  LeftPortType=input  RightPortType=output  PseudoPeriodic=off  Frequencies=[]  VectorFormat=1-D array  Unit=W  AffineConversion=off
  w : PMIOPort  Side=Right
  trq : PMIOPort  Port=2  Side=Right
  Pm_motor : Outport
  tag scope: Pm_motor=global
  wires:
  PS-Simulink Converter3/1 -> " W to kW "/1
  " W to kW "/1 -> Pm_motor/1, [Pm_motor]  "Motor"
  connections:
  PS Product/RConn1 -- PS-Simulink Converter3/LConn1
  PS Product/LConn2 -- w/RConn1
  PS Product/LConn1 -- trq/RConn1
